simulink subsystem "PvtSubSys_VSM_LCK"  (R2020b)
settings: Solver=VariableStepAuto  StartTime=0.0  StopTime=10.0  RelTol=1e-3
values from neighbouring files (symbols this model uses):
  LCK_STATE : value not decoded    [LCK.sldd]
  P_VSM_LCK_A1 = 15.0    [LCK.sldd]
  P_VSM_LCK_AbsEspInTime = 3.0    [LCK.sldd]
  P_VSM_LCK_absLongitudeAccIn = 2.5    [LCK.sldd]
  P_VSM_LCK_absLongitudeAccOut = 3.0    [LCK.sldd]
  P_VSM_LCK_AccRateIn = 30.0    [LCK.sldd]
  P_VSM_LCK_AccRateInTime = 1.5    [LCK.sldd]
  P_VSM_LCK_AccRateOut = 80.0    [LCK.sldd]
  P_VSM_LCK_AccrPelOut = 30.0    [LCK.sldd]
  P_VSM_LCK_AccrPelRateOut = 0.0    [LCK.sldd]
  P_VSM_LCK_BrakePressIn = 3.0    [LCK.sldd]
  P_VSM_LCK_BrakePressInTime = 1.5    [LCK.sldd]
  P_VSM_LCK_BrakePressOut = 5.0    [LCK.sldd]
  P_VSM_LCK_C0 = 0.4    [LCK.sldd]
  P_VSM_LCK_DrvInputTrqValueIn = 2.0    [LCK.sldd]
  P_VSM_LCK_DrvInputTrqValueInTime = 3.0    [LCK.sldd]
  P_VSM_LCK_DrvInputTrqValueOut = 2.3    [LCK.sldd]
  P_VSM_LCK_dypreFactor = 1.0    [LCK.sldd]
  P_VSM_LCK_IdleInTime = 2.0    [LCK.sldd]
  P_VSM_LCK_LanechangeSwitch = 0.0    [LCK.sldd]
  P_VSM_LCK_LaneDouble = 1.0    [LCK.sldd]
  P_VSM_LCK_Lanewidthswitch = 1.0    [LCK.sldd]
  P_VSM_LCK_LateralAcceIn = 3.0    [LCK.sldd]
  P_VSM_LCK_LateralAcceInTime = 3.0    [LCK.sldd]
  P_VSM_LCK_LateralAcceOut = 3.5    [LCK.sldd]
  P_VSM_LCK_LCDrvInputTrqValueOut = 3.0    [LCK.sldd]
  P_VSM_LCK_LCOverrideTime = 0.6    [LCK.sldd]
  P_VSM_LCK_LCOverrideValue = 1.5    [LCK.sldd]
  P_VSM_LCK_LongitudeAccIn = 3.0    [LCK.sldd]
  P_VSM_LCK_LongitudeAccInTime = 3.0    [LCK.sldd]
  P_VSM_LCK_LongitudeAccOut = 3.5    [LCK.sldd]
  P_VSM_LCK_OverrideInTime = 3.0    [LCK.sldd]
  P_VSM_LCK_OverrideTime = 0.3    [LCK.sldd]
  P_VSM_LCK_OverrideValue = 1.2    [LCK.sldd]
  P_VSM_LCK_ParamA1 : value not decoded    [LCK.sldd]
  P_VSM_LCK_PreTime = 0.2    [LCK.sldd]
  P_VSM_LCK_State_Absesp_enable = 1.0    [LCK.sldd]
  P_VSM_LCK_State_Accpedalrate_enable = 0.0    [LCK.sldd]
  P_VSM_LCK_State_Breakpressure_enable = 1.0    [LCK.sldd]
  P_VSM_LCK_State_DriverInputTrqValue_enable = 1.0    [LCK.sldd]
  P_VSM_LCK_State_Eps_enable = 1.0    [LCK.sldd]
  P_VSM_LCK_State_ESSSts_enable = 1.0    [LCK.sldd]
  P_VSM_LCK_State_GEAR_enable = 1.0    [LCK.sldd]
  P_VSM_LCK_State_Handson_enable = 1.0    [LCK.sldd]
  P_VSM_LCK_State_IdleInTime_enable = 0.0    [LCK.sldd]
  P_VSM_LCK_State_Lane_enable = 1.0    [LCK.sldd]
  P_VSM_LCK_State_LaneChange_enable = 1.0    [LCK.sldd]
  P_VSM_LCK_State_LaneCurve_enable = 0.0    [LCK.sldd]
  P_VSM_LCK_State_LateralAcce_enable = 1.0    [LCK.sldd]
  P_VSM_LCK_State_LongitudeAcc_enable = 1.0    [LCK.sldd]
  P_VSM_LCK_State_LSMLine_enable = 1.0    [LCK.sldd]
  P_VSM_LCK_State_Overide_enable = 1.0    [LCK.sldd]
  P_VSM_LCK_State_Param_LaneCurve : value not decoded    [LCK.sldd]
  P_VSM_LCK_State_Param_LaneCurve_Offset : value not decoded    [LCK.sldd]
  P_VSM_LCK_State_Param_LaneWidth : value not decoded    [LCK.sldd]
  P_VSM_LCK_State_Param_LaneWidth_Offset : value not decoded    [LCK.sldd]
  P_VSM_LCK_State_SteerWheelAngle_enable = 1.0    [LCK.sldd]
  P_VSM_LCK_State_SteerWheelSpd_enable = 1.0    [LCK.sldd]
  P_VSM_LCK_State_TargetLaneIn_enable = 1.0    [LCK.sldd]
  P_VSM_LCK_State_TurnLight_enable = 1.0    [LCK.sldd]
  P_VSM_LCK_State_Vehspeed_enable = 1.0    [LCK.sldd]
  P_VSM_LCK_State_Yawsup_enable = 1.0    [LCK.sldd]
  P_VSM_LCK_SteerAngleSpdIn = 150.0    [LCK.sldd]
  P_VSM_LCK_SteerAngleSpdInTime = 3.0    [LCK.sldd]
  P_VSM_LCK_SteerAngleSpdOut = 200.0    [LCK.sldd]
  P_VSM_LCK_SteerWheelAngleIn = 70.0    [LCK.sldd]
  P_VSM_LCK_SteerWheelAngleInTime = 3.0    [LCK.sldd]
  P_VSM_LCK_SteerWheelAngleOut = 90.0    [LCK.sldd]
  P_VSM_LCK_T0 = 0.75    [LCK.sldd]
  P_VSM_LCK_T1 = 15.0    [LCK.sldd]
  P_VSM_LCK_TargetInSwitch = 0.0    [LCK.sldd]
  P_VSM_LCK_Warnarea1 = -0.55    [LCK.sldd]
  P_VSM_LCK_Warnarea2 = -0.35    [LCK.sldd]
  P_VSM_LCK_YawRateIn = 0.2    [LCK.sldd]
  P_VSM_LCK_YawRateInTime = 1.0    [LCK.sldd]
  P_VSM_LCK_YawRateOut = 0.25    [LCK.sldd]
undefined symbols (not defined in the file or in its folder): P_VSM_LSMC_SampleTime
libraries: simulink x275
(part 1 of 5)
settings Model: Creator=GW00133806  LastModifiedBy=GW00201299

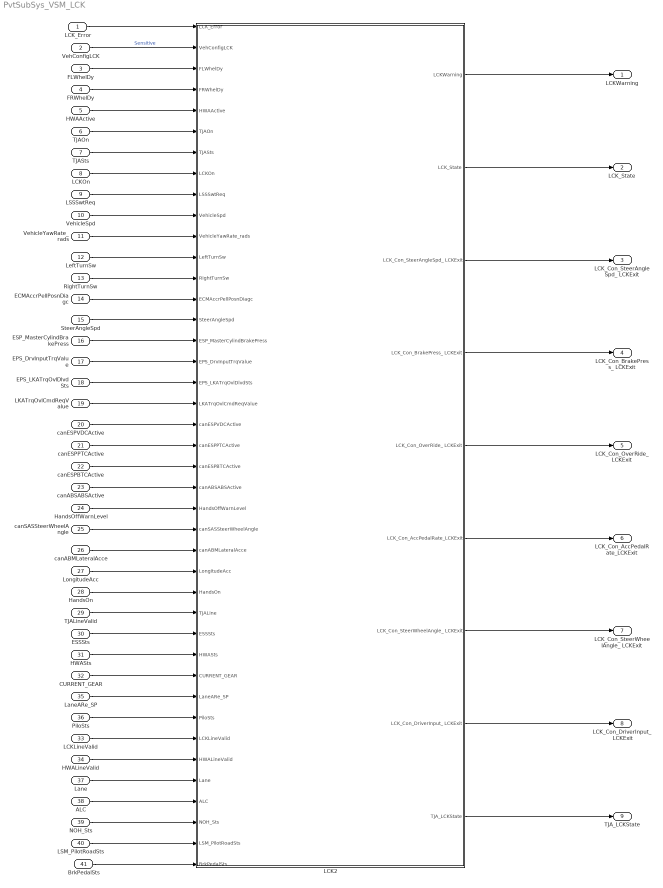
== system PvtSubSys_VSM_LCK ==
  LCK_Error : Inport
  VehConfigLCK : Inport  Port=2  OutDataTypeStr=uint8
  FLWhelDy : Inport  Port=3  OutDataTypeStr=single
  FRWhelDy : Inport  Port=4  OutDataTypeStr=single
  HWAActive : Inport  Port=5  OutDataTypeStr=boolean
  TJAOn : Inport  Port=6  OutDataTypeStr=boolean
  TJASts : Inport  Port=7  OutDataTypeStr=uint8
  LCKOn : Inport  Port=8
  LSSSwtReq : Inport  Port=9
  VehicleSpd : Inport  Port=10  OutDataTypeStr=single
  VehicleYawRate_rads : Inport  Port=11  OutDataTypeStr=single
  LeftTurnSw : Inport  Port=12  OutDataTypeStr=boolean
  RightTurnSw : Inport  Port=13  OutDataTypeStr=boolean
  ECMAccrPellPosnDiagc : Inport  Port=14  OutDataTypeStr=single
  SteerAngleSpd : Inport  Port=15  OutDataTypeStr=single
  ESP_MasterCylindBrakePress : Inport  Port=16  OutDataTypeStr=single
  EPS_DrvInputTrqValue : Inport  Port=17  OutDataTypeStr=single
  EPS_LKATrqOvlDlvdSts : Inport  Port=18  OutDataTypeStr=uint8
  LKATrqOvlCmdReqValue : Inport  Port=19  OutDataTypeStr=single
  canESPVDCActive : Inport  Port=20  OutDataTypeStr=boolean
  canESPPTCActive : Inport  Port=21  OutDataTypeStr=boolean
  canESPBTCActive : Inport  Port=22  OutDataTypeStr=boolean
  canABSABSActive : Inport  Port=23  OutDataTypeStr=boolean
  HandsOffWarnLevel : Inport  Port=24  OutDataTypeStr=uint8
  canSASSteerWheelAngle : Inport  Port=25  OutDataTypeStr=single
  canABMLateralAcce : Inport  Port=26  OutDataTypeStr=single
  LongitudeAcc : Inport  Port=27  OutDataTypeStr=single
  HandsOn : Inport  Port=28  OutDataTypeStr=boolean
  TJALineValid : Inport  Port=29
  ESSSts : Inport  Port=30  OutDataTypeStr=uint8
  HWASts : Inport  Port=31  OutDataTypeStr=uint8
  CURRENT_GEAR : Inport  Port=32  OutDataTypeStr=uint8
  LCKLineValid : Inport  Port=33  OutDataTypeStr=boolean
  HWALineValid : Inport  Port=34
  LaneARe_SP : Inport  Port=35  OutDataTypeStr=Bus: LaneARe_SP_LCK
  PiloSts : Inport  Port=36
  Lane : Inport  Port=37
  ALC : Inport  Port=38
  NOH_Sts : Inport  Port=39
  LSM_PilotRoadSts : Inport  Port=40
  BrkPedalSts : Inport  Port=41
  LCK2 : Subsystem
  LCKWarning : Outport
  LCK_State : Outport  Port=2
  LCK_Con_SteerAngleSpd_ LCKExit : Outport  Port=3
  LCK_Con_BrakePress_ LCKExit : Outport  Port=4
  LCK_Con_OverRide_ LCKExit : Outport  Port=5
  LCK_Con_AccPedalRate_LCKExit : Outport  Port=6
  LCK_Con_SteerWheelAngle_ LCKExit : Outport  Port=7
  LCK_Con_DriverInput_ LCKExit : Outport  Port=8
  TJA_LCKState : Outport  Port=9
  wires:
  LSM_PilotRoadSts/1 -> LCK2/40(LSM_PilotRoadSts)
  NOH_Sts/1 -> LCK2/39(NOH_Sts)
  Lane/1 -> LCK2/37(Lane)
  LeftTurnSw/1 -> LCK2/12(LeftTurnSw)
  LaneARe_SP/1 -> LCK2/33(LaneARe_SP)
  canESPVDCActive/1 -> LCK2/20(canESPVDCActive)
  canABMLateralAcce/1 -> LCK2/26(canABMLateralAcce)
  canSASSteerWheelAngle/1 -> LCK2/25(canSASSteerWheelAngle)
  LCK2/3(LCK_Con_SteerAngleSpd_ LCKExit) -> LCK_Con_SteerAngleSpd_ LCKExit/1
  HandsOn/1 -> LCK2/28(HandsOn)
  PiloSts/1 -> LCK2/34(PiloSts)
  ESP_MasterCylindBrakePress/1 -> LCK2/16(ESP_MasterCylindBrakePress)
  ESSSts/1 -> LCK2/30(ESSSts)
  CURRENT_GEAR/1 -> LCK2/32(CURRENT_GEAR)
  HWASts/1 -> LCK2/31(HWASts)
  canESPBTCActive/1 -> LCK2/22(canESPBTCActive)
  canABSABSActive/1 -> LCK2/23(canABSABSActive)
  HandsOffWarnLevel/1 -> LCK2/24(HandsOffWarnLevel)
  LongitudeAcc/1 -> LCK2/27(LongitudeAcc)
  LKATrqOvlCmdReqValue/1 -> LCK2/19(LKATrqOvlCmdReqValue)
  EPS_DrvInputTrqValue/1 -> LCK2/17(EPS_DrvInputTrqValue)
  SteerAngleSpd/1 -> LCK2/15(SteerAngleSpd)
  FLWhelDy/1 -> LCK2/3(FLWhelDy)
  EPS_LKATrqOvlDlvdSts/1 -> LCK2/18(EPS_LKATrqOvlDlvdSts)
  RightTurnSw/1 -> LCK2/13(RightTurnSw)
  HWAActive/1 -> LCK2/5(HWAActive)
  ECMAccrPellPosnDiagc/1 -> LCK2/14(ECMAccrPellPosnDiagc)
  LCK2/9(TJA_LCKState) -> TJA_LCKState/1
  LCK2/5(LCK_Con_OverRide_ LCKExit) -> LCK_Con_OverRide_ LCKExit/1
  VehicleSpd/1 -> LCK2/10(VehicleSpd)
  LCK2/7(LCK_Con_SteerWheelAngle_ LCKExit) -> LCK_Con_SteerWheelAngle_ LCKExit/1
  LCK2/6(LCK_Con_AccPedalRate_LCKExit) -> LCK_Con_AccPedalRate_LCKExit/1
  VehConfigLCK/1 -> LCK2/2(VehConfigLCK)  "Sensitive"
  VehicleYawRate_rads/1 -> LCK2/11(VehicleYawRate_rads)
  LSSSwtReq/1 -> LCK2/9(LSSSwtReq)
  LCK2/4(LCK_Con_BrakePress_ LCKExit) -> LCK_Con_BrakePress_ LCKExit/1
  LCK2/8(LCK_Con_DriverInput_ LCKExit) -> LCK_Con_DriverInput_ LCKExit/1
  TJALineValid/1 -> LCK2/29(TJALine)
  LCKOn/1 -> LCK2/8(LCKOn)
  LCK2/1(LCKWarning) -> LCKWarning/1
  LCK2/2(LCK_State) -> LCK_State/1
  FRWhelDy/1 -> LCK2/4(FRWhelDy)
  TJASts/1 -> LCK2/7(TJASts)
  LCK_Error/1 -> LCK2/1(LCK_Error)
  TJAOn/1 -> LCK2/6(TJAOn)
  canESPPTCActive/1 -> LCK2/21(canESPPTCActive)
  LCKLineValid/1 -> LCK2/35(LCKLineValid)
  HWALineValid/1 -> LCK2/36(HWALineValid)
  ALC/1 -> LCK2/38(ALC)
  BrkPedalSts/1 -> LCK2/41(BrkPedalSts)

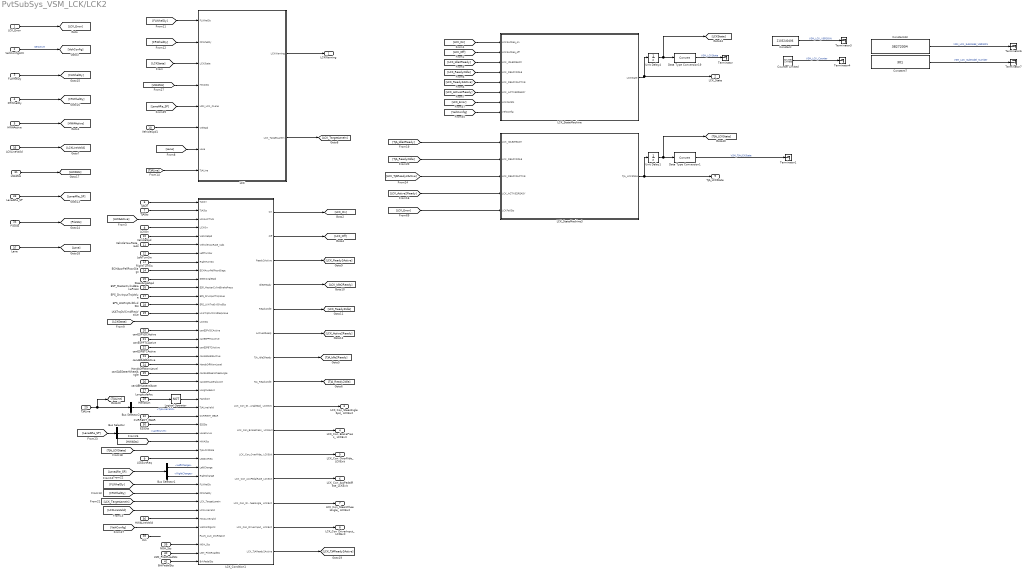
== system PvtSubSys_VSM_LCK/LCK2 ==
  LCK_Error : Inport
  VehConfigLCK : Inport  Port=2  OutDataTypeStr=uint8
  FLWhelDy : Inport  Port=3  OutDataTypeStr=single
  FRWhelDy : Inport  Port=4  OutDataTypeStr=single
  HWAActive : Inport  Port=5  OutDataTypeStr=boolean
  TJAOn : Inport  Port=6  OutDataTypeStr=boolean
  TJASts : Inport  Port=7  OutDataTypeStr=uint8
  LCKOn : Inport  Port=8
  LSSSwtReq : Inport  Port=9
  VehicleSpd : Inport  Port=10  OutDataTypeStr=single
  VehicleYawRate_rads : Inport  Port=11  OutDataTypeStr=single
  LeftTurnSw : Inport  Port=12  OutDataTypeStr=boolean
  RightTurnSw : Inport  Port=13  OutDataTypeStr=boolean
  ECMAccrPellPosnDiagc : Inport  Port=14  OutDataTypeStr=single
  SteerAngleSpd : Inport  Port=15  OutDataTypeStr=single
  ESP_MasterCylindBrakePress : Inport  Port=16  OutDataTypeStr=single
  EPS_DrvInputTrqValue : Inport  Port=17  OutDataTypeStr=single
  EPS_LKATrqOvlDlvdSts : Inport  Port=18  OutDataTypeStr=uint8
  LKATrqOvlCmdReqValue : Inport  Port=19  OutDataTypeStr=single
  canESPVDCActive : Inport  Port=20  OutDataTypeStr=boolean
  canESPPTCActive : Inport  Port=21  OutDataTypeStr=boolean
  canESPBTCActive : Inport  Port=22  OutDataTypeStr=boolean
  canABSABSActive : Inport  Port=23  OutDataTypeStr=boolean
  HandsOffWarnLevel : Inport  Port=24  OutDataTypeStr=uint8
  canSASSteerWheelAngle : Inport  Port=25  OutDataTypeStr=single
  canABMLateralAcce : Inport  Port=26  OutDataTypeStr=single
  LongitudeAcc : Inport  Port=27  OutDataTypeStr=single
  HandsOn : Inport  Port=28  OutDataTypeStr=boolean
  TJALine : Inport  Port=29
  ESSSts : Inport  Port=30  OutDataTypeStr=uint8
  HWASts : Inport  Port=31  OutDataTypeStr=uint8
  CURRENT_GEAR : Inport  Port=32  OutDataTypeStr=uint8
  LaneARe_SP : Inport  Port=33
  PiloSts : Inport  Port=34
  LCKLineValid : Inport  Port=35
  HWALineValid : Inport  Port=36
  Lane : Inport  Port=37
  ALC : Inport  Port=38
  NOH_Sts : Inport  Port=39
  LSM_PilotRoadSts : Inport  Port=40
  BrkPedalSts : Inport  Port=41
  Bus Selector : BusSelector  OutputSignals=LaneCurve
  Bus Selector1 : BusSelector  OutputSignals=LeftChange,RightChange
  Bus Selector2 : BusSelector  OutputSignals=TJALineValid
  Constant : Constant  Value=2103240406  OutDataTypeStr=uint32
  Constant43 : Constant  Value=38272004  OutDataTypeStr=uint32
  Constant7 : Constant  Value=301  OutDataTypeStr=uint16
  Counter Limited : simulink/Sources/Counter Limited  uplimit=7  tsamp=-1
  Data Type Conversion1 : DataTypeConversion
  Data Type Conversion19 : DataTypeConversion
  LCK : Subsystem
  LCK_Condition1 : Subsystem
  LCK_StateMachine : Subsystem
  LCK_StateMachine3 : Subsystem
  Logical Operator : Logic  Operator=NOT  AllPortsSameDT=off  OutDataTypeStr=boolean
  Terminator{,1,3..4,6..7} (6 alike) : Terminator
  Unit Delay1 : UnitDelay  InitialCondition=LCK_STATE.LCK_Off  SampleTime=-1  HasFrameUpgradeWarning=on
  Unit Delay4 : UnitDelay  InitialCondition=LCK_STATE.LCK_Off  SampleTime=-1  HasFrameUpgradeWarning=on
  VehicleSpd1 : InportShadow  Port=10  OutDataTypeStr=single
  LCKWarning : Outport
  LCK_State : Outport  Port=2
  LCK_Con_SteerAngleSpd_ LCKExit : Outport  Port=3
  LCK_Con_BrakePress_ LCKExit : Outport  Port=4
  LCK_Con_OverRide_ LCKExit : Outport  Port=5
  LCK_Con_AccPedalRate_LCKExit : Outport  Port=6
  LCK_Con_SteerWheelAngle_ LCKExit : Outport  Port=7
  LCK_Con_DriverInput_ LCKExit : Outport  Port=8
  TJA_LCKState : Outport  Port=9
  wires:
  BrkPedalSts/1 -> LCK_Condition1/43(BrkPedalSts)
  ALC/1 -> ?
  HWASts/1 -> [HWASts]
  VehicleSpd1/1 -> LCK/6(VehSpd)
  LCK/2(LCK_TargetLaneIn) -> [LCK_TargetLaneIn]
  [VehConfig] -> LCK_Condition1/39(VehConfigLCK)
  HWALineValid/1 -> LCK_Condition1/38(HWALineValid)
  [LCKLineValid] -> LCK_Condition1/37(LCKLineValid)
  [LCK_TargetLaneIn] -> LCK_Condition1/36(LCK_TargetLaneIn)
  Counter Limited/1 -> Terminator4/1  "VSM_LCK_Counter"
  Constant/1 -> Terminator3/1  "VSM_LCK_VERSION"
  Logical Operator/1 -> LCK_Condition1/24(HandsOn)
  LCKLineValid/1 -> [LCKLineValid]
  LCK_Condition1/1(On) -> [LCK_On]
  LCK_Condition1/7(TJA_Idle2Ready) -> [TJA_Idle2Ready]
  LCK_Condition1/8(TJA_Ready2Idle) -> [TJA_Ready2Idle]
  [HWAActive] -> LCK_Condition1/3(HWAACTIVE)
  [LCK_Ready2Active] -> LCK_StateMachine/5(LCK_READY2ACTIVE)
  LCK_Condition1/2(Off) -> [LCK_Off]
  Data Type Conversion1/1 -> Terminator1/1  "VSM_TJALCKState"
  [TJA_LCKState] -> LCK_Condition1/30(TJALCKState)
  RightTurnSw/1 -> LCK_Condition1/8(RightTurnSw)
  LSSSwtReq/1 -> LCK_Condition1/31(LSSSwtReq)
  VehicleYawRate_rads/1 -> LCK_Condition1/6(VehicleYawRate_rads)
  [LCKState] -> LCK_Condition1/15(LCKSts)
  Data Type Conversion19/1 -> Terminator/1  "VSM_LCKState"
  LCK_StateMachine3/1(TJA_LCKState) -> Unit Delay1/1, TJA_LCKState/1
  Bus Selector/1 -> LCK_Condition1/28(LaneCurve)  "<LaneCurve>"
  [LCK_TJAReady2Active] -> LCK_StateMachine3/3(LCK_READY2ACTIVE)
  LCK_Condition1/4(Idle2Ready) -> [LCK_Idle2Ready]
  LaneARe_SP/1 -> [LaneARe_SP]
  [TJA_Idle2Ready] -> LCK_StateMachine3/1(LCK_IDLE2READY)
  SteerAngleSpd/1 -> LCK_Condition1/10(SteerAngleSpd)
  [TJA_Ready2Idle] -> LCK_StateMachine3/2(LCK_READY2IDLE)
  ESP_MasterCylindBrakePress/1 -> LCK_Condition1/11(ESP_MasterCylindBrakePress)
  [LCK_Off] -> LCK_StateMachine/2(LCKSwtReq_off)
  ECMAccrPellPosnDiagc/1 -> LCK_Condition1/9(ECMAccrPellPosnDiagc)
  HandsOffWarnLevel/1 -> LCK_Condition1/20(HandsOffWarnLevel)
  EPS_DrvInputTrqValue/1 -> LCK_Condition1/12(EPS_DrvInputTrqValue)
  canSASSteerWheelAngle/1 -> LCK_Condition1/21(canSASSteerWheelAngle)
  LCK_Condition1/10(LCK_Con_BrakePress_ LCKExit) -> LCK_Con_BrakePress_ LCKExit/1
  canABSABSActive/1 -> LCK_Condition1/19(canABSABSActive)
  [FLWhelDy] -> LCK_Condition1/34(FLWhelDy)
  Unit Delay1/1 -> [TJA_LCKState], Data Type Conversion1/1
  EPS_LKATrqOvlDlvdSts/1 -> LCK_Condition1/13(EPS_LKATrqOvlDlvdSts)
  TJASts/1 -> LCK_Condition1/2(TJASts)
  [FLWhelDy] -> LCK/1(FLWhelDy)
  [VehConfig] -> LCK_StateMachine/8(VehConfig)
  LCK_Condition1/9(LCK_Con_SteerAngleSpd_ LCKExit) -> LCK_Con_SteerAngleSpd_ LCKExit/1
  FLWhelDy/1 -> [FLWhelDy]
  canABMLateralAcce/1 -> LCK_Condition1/22(canABMLateralAcce)
  CURRENT_GEAR/1 -> LCK_Condition1/26(CURRENT_GEAR)
  LCK_StateMachine/1(LCKState) -> LCK_State/1, Unit Delay4/1
  LKATrqOvlCmdReqValue/1 -> LCK_Condition1/14(LKATrqOvlCmdReqValue)
  LCKOn/1 -> LCK_Condition1/4(LCKOn)
  [LCK_Ready2Idle] -> LCK_StateMachine/4(LCK_READY2IDLE)
  canESPBTCActive/1 -> LCK_Condition1/18(canESPBTCActive)
  LCK/1(LCKWarning) -> LCKWarning/1
  [HWASts] -> LCK_Condition1/29(HWASts)
  LCK_Condition1/12(LCK_Con_AccPedalRate_LCKExit) -> LCK_Con_AccPedalRate_LCKExit/1
  LCK_Condition1/14(LCK_Con_DriverInput_ LCKExit) -> LCK_Con_DriverInput_ LCKExit/1
  LCK_Condition1/6(Active2Ready) -> [LCK_Active2Ready]
  LongitudeAcc/1 -> LCK_Condition1/23(LongitudeAcc)
  TJAOn/1 -> LCK_Condition1/1(TJAOn)
  LeftTurnSw/1 -> LCK_Condition1/7(LeftTurnSw)
  [FRWhelDy] -> LCK_Condition1/35(FRWhelDy)
  [LCK_On] -> LCK_StateMachine/1(LCKSwtReq_on)
  canESPVDCActive/1 -> LCK_Condition1/16(canESPVDCActive)
  HWAActive/1 -> [HWAActive]
  ESSSts/1 -> LCK_Condition1/27(ESSSts)
  [LCK_Error] -> LCK_StateMachine3/5(LCKFailSts)
  [LCKState] -> LCK/3(LCKState)
  LCK_Error/1 -> [LCK_Error]
  HandsOn/1 -> Logical Operator/1
  [LCK_Active2Ready] -> LCK_StateMachine/6(LCK_ACTIVE2READY)
  [HWASts] -> LCK/4(HWASts)
  LCK_Condition1/11(LCK_Con_OverRide_ LCKExit) -> LCK_Con_OverRide_ LCKExit/1
  VehicleSpd/1 -> LCK_Condition1/5(VehicleSpd)
  PiloSts/1 -> [PiloSts]
  [LCK_Active2Ready] -> LCK_StateMachine3/4(LCK_ACTIVE2READY)
  [FRWhelDy] -> LCK/2(FRWhelDy)
  [LCK_Idle2Ready] -> LCK_StateMachine/3(LCK_IDLE2READY)
  LCK_Condition1/13(LCK_Con_SteerWheelAngle_ LCKExit) -> LCK_Con_SteerWheelAngle_ LCKExit/1
  [LCK_Error] -> LCK_StateMachine/7(LCKFailSts)
  FRWhelDy/1 -> [FRWhelDy]
  canESPPTCActive/1 -> LCK_Condition1/17(canESPPTCActive)
  LCK_Condition1/5(Ready2Idle) -> [LCK_Ready2Idle]
  VehConfigLCK/1 -> [VehConfig]  "Sensitive"
  Unit Delay4/1 -> [LCKState], Data Type Conversion19/1
  LCK_Condition1/3(Ready2Active) -> [LCK_Ready2Active]
  [LaneARe_SP] -> Bus Selector/1
  [LaneARe_SP] -> LCK/5(LSM_LCK_CLane)
  Lane/1 -> [Lane]
  [Lane] -> LCK/7(Lane)
  Constant43/1 -> Terminator6/1  "VSM_LCK_SubModel_VERSION"
  Constant7/1 -> Terminator7/1  "VSM_LCK_SubModel_Number"
  [LaneARe_SP] -> Bus Selector1/1
  Bus Selector1/1 -> LCK_Condition1/32(LeftChange)  "<LeftChange>"
  Bus Selector1/2 -> LCK_Condition1/33(RightChange)  "<RightChange>"
  NOH_Sts/1 -> LCK_Condition1/41(NOH_Sts)
  LSM_PilotRoadSts/1 -> LCK_Condition1/42(LSM_PilotRoadSts)
  LCK_Condition1/15(LCK_TJAReady2Active) -> [LCK_TJAReady2Active]
  TJALine/1 -> [TJALine], Bus Selector2/1
  Bus Selector2/1 -> LCK_Condition1/25(TJALineValid)  "<TJALineValid>"
  [TJALine] -> LCK/8(TJALine)
